simulink model "IPCore_3Level_PWM"  (R2024a)
settings: Solver=VariableStepAuto  StartTime=0.0  StopTime=0.001  RelTol=1e-3
values from neighbouring files (symbols this model uses):
  f_FPGA_clk = 100e6    (= 100000000)    [Init_IP_Core.m]
  T_FPGA_clk = 1/f_FPGA_clk    (= 1e-08)    [Init_IP_Core.m]
libraries: hdlsllib x1
settings Model: PacingRate=0.000100  Creator=info  LastModifiedBy=info

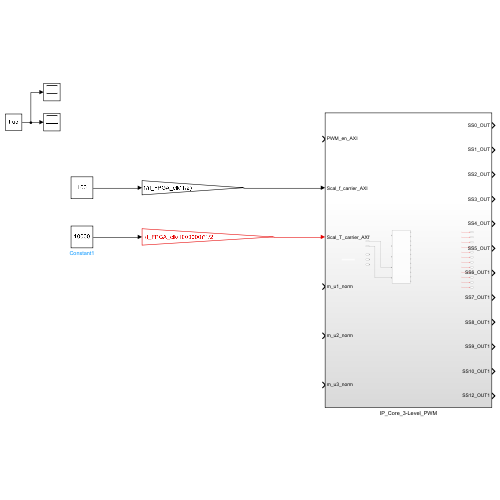
[thumbnail: Simulink's stored preview of the top-level diagram]
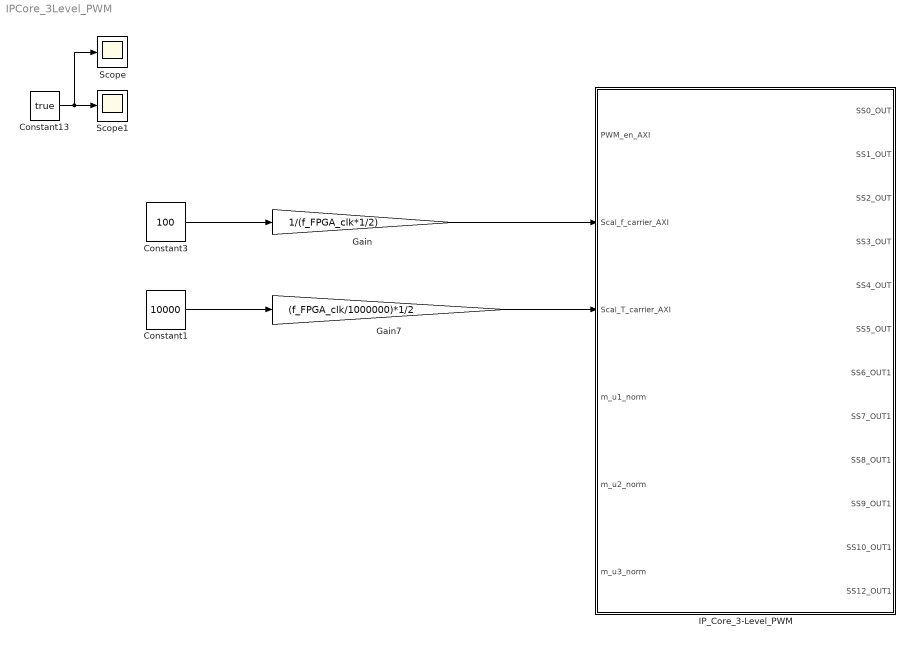
== system IPCore_3Level_PWM ==
  Constant1 : Constant  Value=10000  SampleTime=f_FPGA_clk
  Constant13 : Constant  Value=true  SampleTime=T_FPGA_clk
  Constant3 : Constant  Value=100  SampleTime=f_FPGA_clk
  Gain : Gain  Gain=1/(f_FPGA_clk*1/2)  OutDataTypeStr=fixdt(0,25,26)
  Gain7 : Gain  Gain=(f_FPGA_clk/1000000)*1/2  OutDataTypeStr=fixdt(0,25,0)
  IP_Core_3-Level_PWM : Subsystem
  Scope : Scope
  Scope1 : Scope
  wires:
  Gain/1 -> IP_Core_3-Level_PWM/2(Scal_f_carrier_AXI)
  Constant1/1 -> Gain7/1
  Constant3/1 -> Gain/1
  Gain7/1 -> IP_Core_3-Level_PWM/3(Scal_T_carrier_AXI)
  Constant13/1 -> Scope/1, Scope1/1

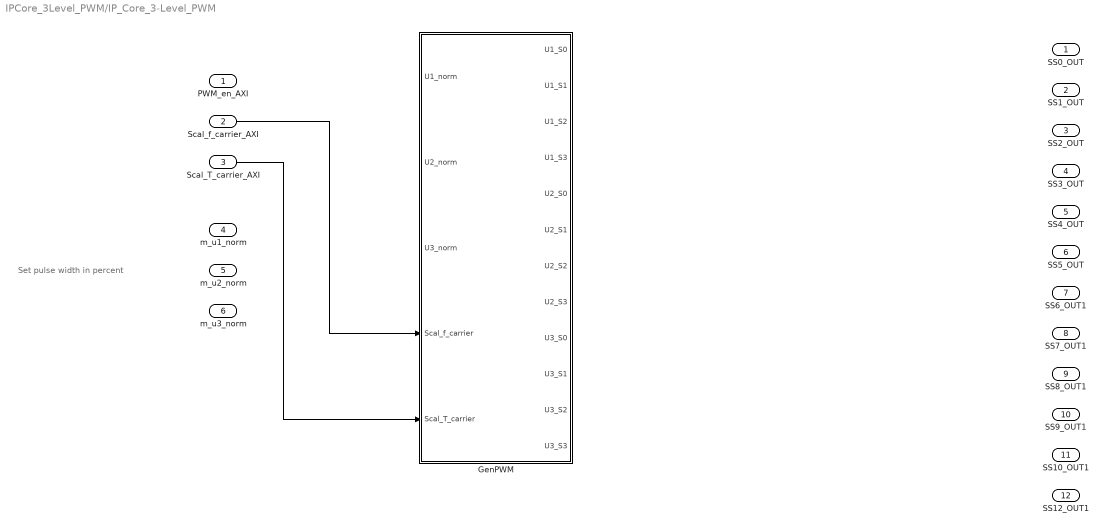
== system IPCore_3Level_PWM/IP_Core_3-Level_PWM ==
  note: Set pulse width in percent
  PWM_en_AXI : Inport
  Scal_f_carrier_AXI : Inport  Port=2
  Scal_T_carrier_AXI : Inport  Port=3
  m_u1_norm : Inport  Port=4
  m_u2_norm : Inport  Port=5
  m_u3_norm : Inport  Port=6
  GenPWM : Subsystem
  SS0_OUT : Outport  VectorParamsAs1DForOutWhenUnconnected=off
  SS1_OUT : Outport  Port=2  VectorParamsAs1DForOutWhenUnconnected=off
  SS2_OUT : Outport  Port=3  VectorParamsAs1DForOutWhenUnconnected=off
  SS3_OUT : Outport  Port=4  VectorParamsAs1DForOutWhenUnconnected=off
  SS4_OUT : Outport  Port=5  VectorParamsAs1DForOutWhenUnconnected=off
  SS5_OUT : Outport  Port=6  VectorParamsAs1DForOutWhenUnconnected=off
  SS6_OUT1 : Outport  Port=7  VectorParamsAs1DForOutWhenUnconnected=off
  SS7_OUT1 : Outport  Port=8  VectorParamsAs1DForOutWhenUnconnected=off
  SS8_OUT1 : Outport  Port=9  VectorParamsAs1DForOutWhenUnconnected=off
  SS9_OUT1 : Outport  Port=10  VectorParamsAs1DForOutWhenUnconnected=off
  SS10_OUT1 : Outport  Port=11  VectorParamsAs1DForOutWhenUnconnected=off
  SS12_OUT1 : Outport  Port=12  VectorParamsAs1DForOutWhenUnconnected=off
  wires:
  ? -> SS1_OUT/1
  ? -> SS5_OUT/1
  ? -> SS3_OUT/1
  ? -> SS2_OUT/1
  ? -> SS0_OUT/1
  ? -> SS4_OUT/1
  ? -> SS7_OUT1/1
  ? -> SS12_OUT1/1
  ? -> SS9_OUT1/1
  ? -> SS8_OUT1/1
  ? -> SS6_OUT1/1
  ? -> SS10_OUT1/1
  Scal_f_carrier_AXI/1 -> GenPWM/4(Scal_f_carrier)
  Scal_T_carrier_AXI/1 -> GenPWM/5(Scal_T_carrier)

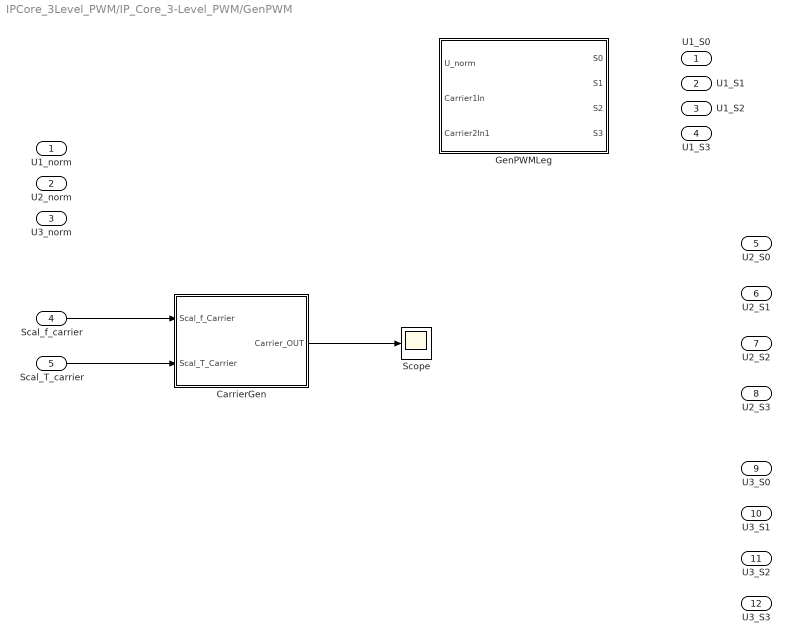
== system IPCore_3Level_PWM/IP_Core_3-Level_PWM/GenPWM ==
  U1_norm : Inport
  U2_norm : Inport  Port=2
  U3_norm : Inport  Port=3
  Scal_f_carrier : Inport  Port=4
  Scal_T_carrier : Inport  Port=5
  CarrierGen : Subsystem
  GenPWMLeg : Subsystem
  Scope : Scope
  U1_S0 : Outport
  U1_S1 : Outport  Port=2
  U1_S2 : Outport  Port=3
  U1_S3 : Outport  Port=4
  U2_S0 : Outport  Port=5
  U2_S1 : Outport  Port=6
  U2_S2 : Outport  Port=7
  U2_S3 : Outport  Port=8
  U3_S0 : Outport  Port=9
  U3_S1 : Outport  Port=10
  U3_S2 : Outport  Port=11
  U3_S3 : Outport  Port=12
  wires:
  Scal_T_carrier/1 -> CarrierGen/2(Scal_T_Carrier)
  Scal_f_carrier/1 -> CarrierGen/1(Scal_f_Carrier)
  CarrierGen/1(Carrier_OUT) -> Scope/1

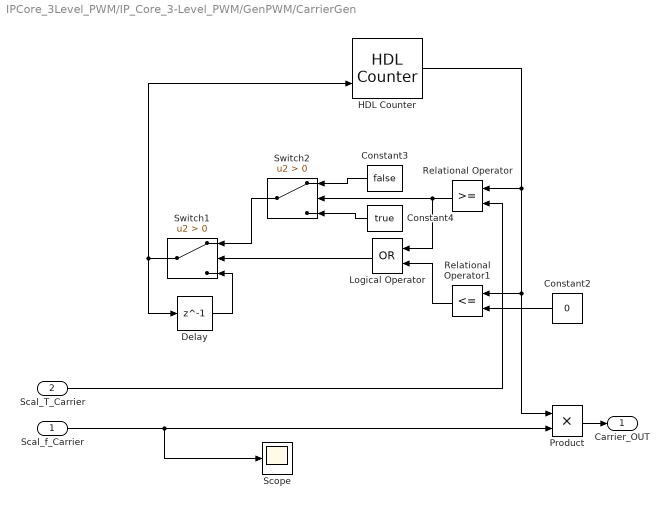
== system IPCore_3Level_PWM/IP_Core_3-Level_PWM/GenPWM/CarrierGen ==
  Scal_f_Carrier : Inport
  Scal_T_Carrier : Inport  Port=2
  Constant2 : Constant  Value=0  SampleTime=f_FPGA_clk
  Constant3 : Constant  Value=false  SampleTime=f_FPGA_clk
  Constant4 : Constant  Value=true  SampleTime=f_FPGA_clk
  Delay : Delay  DelayLength=1
  HDL Counter : hdlsllib/Sources/HDL Counter  CountType=Free running  CountInit=0  CountStep=1  CountMax=25  CountFromType=Initial value  CountFrom=0  CountResetPort=on  CountLoadPort=off  CountEnbPort=off  CountDirPort=on  CountHitOutputPort=off  CountDataType=Unsigned  CountWordLen=20  CountFracLen=0  CountSampTime=1
  Logical Operator : Logic  Operator=OR  AllPortsSameDT=off  OutDataTypeStr=boolean
  Product : Product  OutDataTypeStr=fixdt(0,18,17)
  Relational Operator : RelationalOperator  OutDataTypeStr=boolean  RndMeth=Simplest  InputSameDT=off
  Relational Operator1 : RelationalOperator  Operator=<=  OutDataTypeStr=boolean  RndMeth=Simplest  InputSameDT=off
  Scope : Scope
  Switch1 : Switch  Criteria=u2 > Threshold  SaturateOnIntegerOverflow=off  InputSameDT=off
  Switch2 : Switch  Criteria=u2 > Threshold  SaturateOnIntegerOverflow=off  InputSameDT=off
  Carrier_OUT : Outport
  wires:
  Scal_T_Carrier/1 -> Relational Operator/2
  HDL Counter/1 -> Product/1, Relational Operator1/1, Relational Operator/1
  Constant2/1 -> Relational Operator1/2
  Switch1/1 -> HDL Counter/2, Delay/1
  Relational Operator/1 -> Logical Operator/1, Switch2/2
  Relational Operator1/1 -> Logical Operator/2
  Logical Operator/1 -> Switch1/2
  Delay/1 -> Switch1/3
  Switch2/1 -> Switch1/1
  Constant3/1 -> Switch2/1
  Constant4/1 -> Switch2/3
  Scal_f_Carrier/1 -> Scope/1, Product/2
  Product/1 -> Carrier_OUT/1

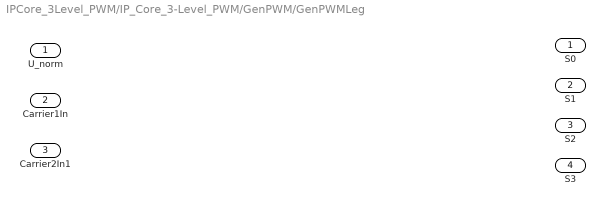
== system IPCore_3Level_PWM/IP_Core_3-Level_PWM/GenPWM/GenPWMLeg ==
  U_norm : Inport
  Carrier1In : Inport  Port=2
  Carrier2In1 : Inport  Port=3
  S0 : Outport
  S1 : Outport  Port=2
  S2 : Outport  Port=3
  S3 : Outport  Port=4
